simulink model "sygyz351"  (R2022a)
settings: Solver=VariableStepAuto  StartTime=0.0  StopTime=200  RelTol=1e-3
settings Model: Creator=dell  LastModifiedBy=dell

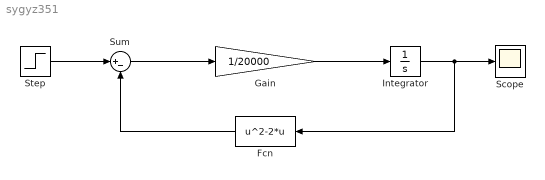
== system sygyz351 ==
  Fcn : Fcn  Expr=u^2-2*u
  Gain : Gain  Gain=1/20000
  Integrator : Integrator
  Scope : Scope
  Step : Step  Time=0  After=150000  SampleTime=0
  Sum : Sum  Inputs=|+-
  wires:
  Step/1 -> Sum/1
  Sum/1 -> Gain/1
  Gain/1 -> Integrator/1
  Integrator/1 -> Fcn/1, Scope/1
  Fcn/1 -> Sum/2
